simulink library "libc_control"  (R2013b)
settings: Solver=FixedStepDiscrete  StartTime=0.0  StopTime=Inf  FixedStep=0.004  RelTol=1e-3
PostLoadFcn:
  | , if any(exist('dsrtsu_mdlpostloadfcn', 'file') == [2, 3, 6]), try dsrtsu_mdlpostloadfcn('Execute', bdroot); catch fprintf('Error in PostLoadFcn (dsrtsu_mdlpostloadfcn) for model "%s":\n %s\n', bdroot, lasterr); end, end,
undefined symbols (not defined in the file or in its folder): DiscIntNeverNeededParam, tA
settings Model: DSRTSU_INTERNAL_RTI_VER=440  DSRTSU_INTERNAL_RTI_TYPE=rti1005  DSRTSU_INTERNAL_RTIFPGA=30  Creator=Falkenhahn  LastModifiedBy=fav

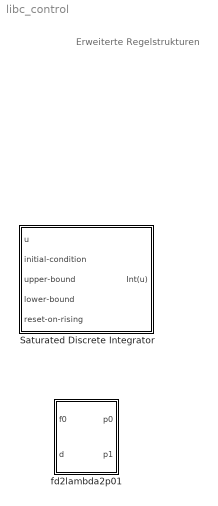
== system libc_control ==
  note: Erweiterte
      | Regelstrukturen
  Saturated Discrete Integrator : Subsystem
  fd2lambda2p01 : MATLAB Function  TreatAsAtomicUnit=on

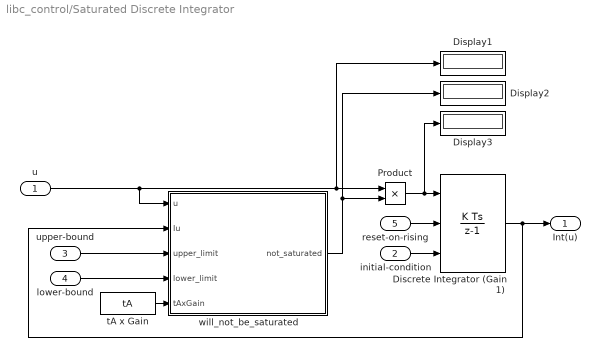
== system libc_control/Saturated Discrete Integrator ==
  u : Inport
  initial-condition : Inport  Port=2
  upper-bound : Inport  Port=3
  lower-bound : Inport  Port=4
  reset-on-rising : Inport  Port=5
  Discrete Integrator (Gain 1) : DiscreteIntegrator  ExternalReset=rising  InitialConditionSource=external  SampleTime=tA  UpperSaturationLimit=0.2  LowerSaturationLimit=-0.1  ICPrevOutput=DiscIntNeverNeededParam  ICPrevScaledInput=DiscIntNeverNeededParam
  Display1 : Display
  Display2 : Display
  Display3 : Display
  Product : Product  RndMeth=Zero
  tA x Gain : Constant  Value=tA
  will_not_be_saturated : MATLAB Function  TreatAsAtomicUnit=on
  Int(u) : Outport
  wires:
  u/1 -> Display1/1, Product/1, will_not_be_saturated/1(u)
  Discrete Integrator (Gain 1)/1 -> will_not_be_saturated/2(Iu), Int(u)/1
  Product/1 -> Display3/1, Discrete Integrator (Gain 1)/1
  will_not_be_saturated/1(not_saturated) -> Display2/1, Product/2
  upper-bound/1 -> will_not_be_saturated/3(upper_limit)
  lower-bound/1 -> will_not_be_saturated/4(lower_limit)
  tA x Gain/1 -> will_not_be_saturated/5(tAxGain)
  reset-on-rising/1 -> Discrete Integrator (Gain 1)/2
  initial-condition/1 -> Discrete Integrator (Gain 1)/3

== matlab function libc_control/Saturated Discrete Integrator/will_not_be_saturated ==
  data: u input; not_saturated output; Iu input; upper_limit input; lower_limit input; tAxGain input
function not_saturated = fcn(u, Iu, upper_limit, lower_limit, tAxGain)

not_saturated = 1;

utAx = u*tAxGain;

if Iu > upper_limit
    not_saturated = 0;
elseif Iu + utAx > upper_limit
    not_saturated = (upper_limit - Iu)/(utAx);
end

if Iu < lower_limit
    not_saturated = 0;
elseif Iu + utAx < lower_limit
    not_saturated = (lower_limit - Iu)/(utAx);
end

== matlab function libc_control/fd2lambda2p01 ==
  data: f0 input; p0 output; d input; p1 output
function [p0, p1] = chcoeffs(f0,d)
%#codegen


w0 = f0*pi*2;

p0 = w0.^2;
p1 = 2*w0.*d;
